simulink model "LugRStEnCtrl"  (R2018b)
settings: Solver=FixedStepDiscrete  StartTime=0.0  StopTime=10.0  FixedStep=0.01  RelTol=1e-3
undefined symbols (not defined in the file or in its folder): data, ThdRwRtStBkReclnEn_Clear, ThdRwRtStBkReclnEn_Set, ThdRwRtStCshnFldEn_Clear, ThdRwRtStCshnFldEn_Set, ThdRwRtStFwdBkwdEn_Clear, ThdRwRtStFwdBkwdEn_Set
libraries: simulink x1
settings Model: Creator=sn2xws  LastModifiedBy=sn2xws
settings DataIOCC: SaveFormat=StructureWithTime
settings OptimizationCC: DefaultParameterBehavior=Inlined  EnhancedBackFolding=on  PassReuseOutputArgsAs=Individual arguments  ZeroExternalMemoryAtStartup=off  ZeroInternalMemoryAtStartup=off  OptimizeBlockOrder=speed  DifferentSizesBufferReuse=on  OptimizationCustomize=off
settings DebuggingCC: ParameterTunabilityLossMsg=error
settings ModelReferenceCC: ModelReferenceNumInstancesAllowed=Single
settings SFSimCC: MATLABDynamicMemAlloc=off
settings RTWCC: SystemTargetFile=autosar.tlc  GenCodeOnly=on  TemplateMakefile=ert_default_tmf  Description=AUTOSAR  GenerateReport=on  IncludeHyperlinkInReport=on  LaunchReport=on  GenerateTraceInfo=on  GenerateTraceReport=on  GenerateTraceReportSl=on  GenerateTraceReportSf=on  GenerateTraceReportEml=on  GenerateCodeMetricsReport=on
settings CodeAppCC: ForceParamTrailComments=on  IgnoreCustomStorageClasses=off  OperatorAnnotations=on  SimulinkDataObjDesc=on  SFDataObjDesc=on  InsertBlockDesc=on
settings STFCustomTargetCC: TargetLangStandard=C99 (ISO)  MultiwordLength=256  ParMdlRefBuildCompliant=on  CompOptLevelCompliant=on  IncludeMdlTerminateFcn=off  CombineOutputUpdateFcns=on  SuppressErrorStatus=on  ERTCustomFileBanners=on  SupportNonFinite=off  SupportComplex=off  SupportContinuousTime=off  SupportNonInlinedSFcns=off  RemoveResetFunc=on  MATLABClassNameForMDSCustomization=Simulink.SoftwareTarget.ERTCustomization  AutosarCompliant=on  UseToolchainInfoCompliant=on  LookupTableObjectStructAxisOrder=2,1,3,4,...  LUTObjectStructOrderEvenSpacing=Size,Table,Breakpoints  SystemTargetFile=autosar.tlc
settings ERTTargetCC: TargetLangStandard=C99 (ISO)  ConcurrentExecutionCompliant=off  IncludeMdlTerminateFcn=off  SuppressErrorStatus=on  SupportNonFinite=off  SupportComplex=off  ModelStepFunctionPrototypeControlCompliant=off  CPPClassGenCompliant=off  AutosarCompliant=on  LookupTableObjectStructAxisOrder=2,1,3,4,...  LUTObjectStructOrderEvenSpacing=Size,Table,Breakpoints  InlinedParameterPlacement=NonHierarchical  ERTCustomFileTemplate=example_file_process.tlc  ERTFilePackagingFormat=Compact

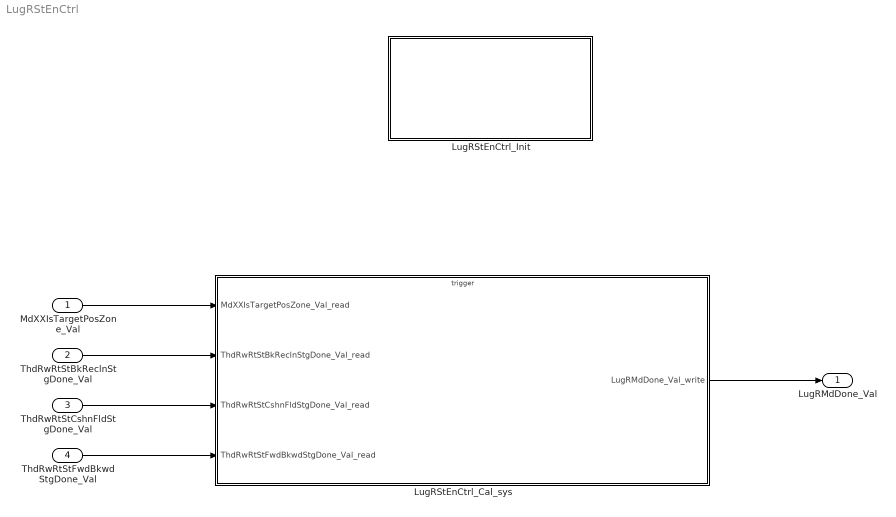
== system LugRStEnCtrl ==
  MdXXIsTargetPosZone_Val : Inport  OutDataTypeStr=uint32  PortDimensions=1
  ThdRwRtStBkReclnStgDone_Val : Inport  Port=2  OutDataTypeStr=boolean  PortDimensions=1
  ThdRwRtStCshnFldStgDone_Val : Inport  Port=3  OutDataTypeStr=boolean  PortDimensions=1
  ThdRwRtStFwdBkwdStgDone_Val : Inport  Port=4  OutDataTypeStr=boolean  PortDimensions=1
  LugRStEnCtrl_Cal_sys : Subsystem
  LugRStEnCtrl_Init : Subsystem
  LugRMdDone_Val : Outport  OutDataTypeStr=uint8  PortDimensions=1
  wires:
  MdXXIsTargetPosZone_Val/1 -> LugRStEnCtrl_Cal_sys/1(MdXXIsTargetPosZone_Val_read)
  ThdRwRtStBkReclnStgDone_Val/1 -> LugRStEnCtrl_Cal_sys/2(ThdRwRtStBkReclnStgDone_Val_read)
  ThdRwRtStCshnFldStgDone_Val/1 -> LugRStEnCtrl_Cal_sys/3(ThdRwRtStCshnFldStgDone_Val_read)
  ThdRwRtStFwdBkwdStgDone_Val/1 -> LugRStEnCtrl_Cal_sys/4(ThdRwRtStFwdBkwdStgDone_Val_read)
  LugRStEnCtrl_Cal_sys/1(LugRMdDone_Val_write) -> LugRMdDone_Val/1

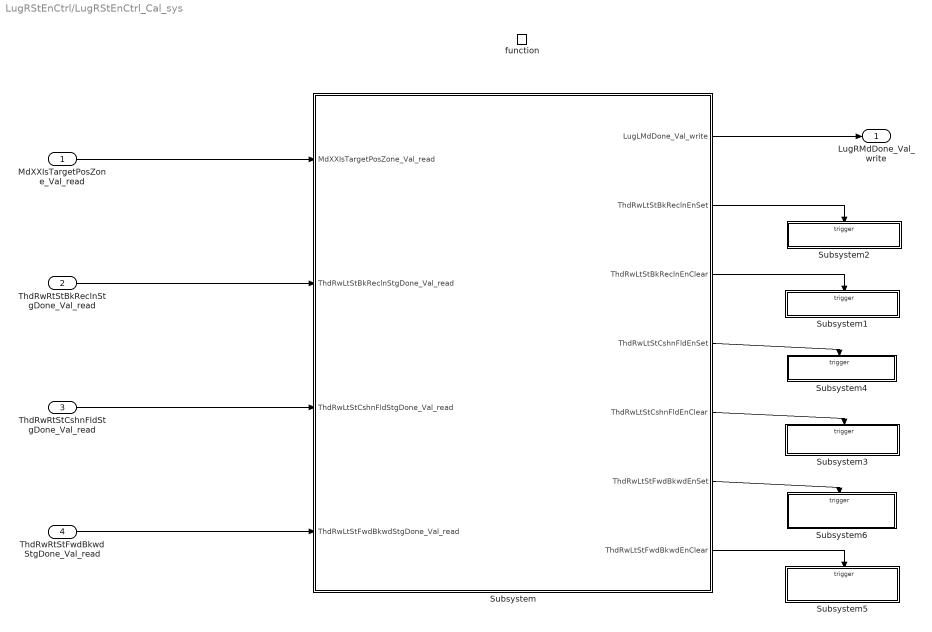
== system LugRStEnCtrl/LugRStEnCtrl_Cal_sys ==
  MdXXIsTargetPosZone_Val_read : Inport
  ThdRwRtStBkReclnStgDone_Val_read : Inport  Port=2
  ThdRwRtStCshnFldStgDone_Val_read : Inport  Port=3
  ThdRwRtStFwdBkwdStgDone_Val_read : Inport  Port=4
  function : TriggerPort  TriggerType=function-call  IsSimulinkFunction=on  FunctionName=LugRStEnCtrl_Cal  VariantControl=(inherit)
  Subsystem : Subsystem
  Subsystem1 : Subsystem
  Subsystem2 : Subsystem
  Subsystem3 : Subsystem
  Subsystem4 : Subsystem
  Subsystem5 : Subsystem
  Subsystem6 : Subsystem
  LugRMdDone_Val_write : Outport
      settings: EnsureOutportIsVirtual=on
  wires:
  Subsystem/7(ThdRwLtStFwdBkwdEnClear) -> Subsystem5/Trigger
  Subsystem/6(ThdRwLtStFwdBkwdEnSet) -> Subsystem6/Trigger
  Subsystem/4(ThdRwLtStCshnFldEnSet) -> Subsystem4/Trigger
  Subsystem/3(ThdRwLtStBkReclnEnClear) -> Subsystem1/Trigger
  Subsystem/2(ThdRwLtStBkReclnEnSet) -> Subsystem2/Trigger
  Subsystem/5(ThdRwLtStCshnFldEnClear) -> Subsystem3/Trigger
  Subsystem/1(LugLMdDone_Val_write) -> LugRMdDone_Val_write/1
  MdXXIsTargetPosZone_Val_read/1 -> Subsystem/1(MdXXIsTargetPosZone_Val_read)
  ThdRwRtStBkReclnStgDone_Val_read/1 -> Subsystem/2(ThdRwLtStBkReclnStgDone_Val_read)
  ThdRwRtStFwdBkwdStgDone_Val_read/1 -> Subsystem/4(ThdRwLtStFwdBkwdStgDone_Val_read)
  ThdRwRtStCshnFldStgDone_Val_read/1 -> Subsystem/3(ThdRwLtStCshnFldStgDone_Val_read)

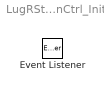
== system LugRStEnCtrl/LugRStEnCtrl_Init ==
  Event Listener : EventListener  EventName=reset

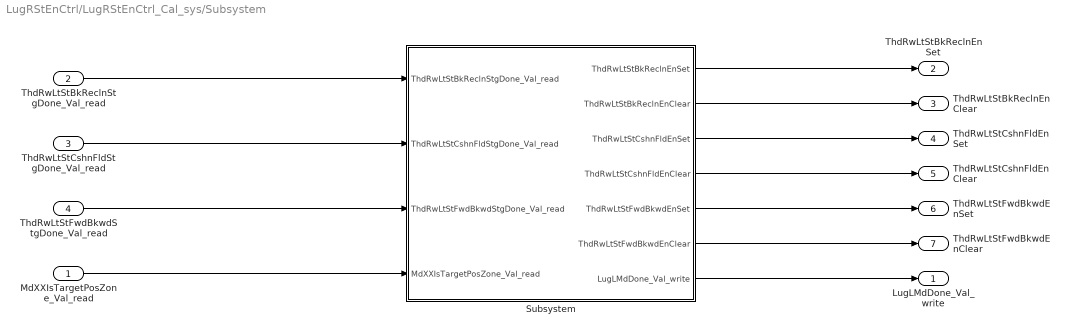
== system LugRStEnCtrl/LugRStEnCtrl_Cal_sys/Subsystem ==
  MdXXIsTargetPosZone_Val_read : Inport
  ThdRwLtStBkReclnStgDone_Val_read : Inport  Port=2
  ThdRwLtStCshnFldStgDone_Val_read : Inport  Port=3
  ThdRwLtStFwdBkwdStgDone_Val_read : Inport  Port=4
  Subsystem : Subsystem
  LugLMdDone_Val_write : Outport
      settings: EnsureOutportIsVirtual=on
  ThdRwLtStBkReclnEnSet : Outport  Port=2
  ThdRwLtStBkReclnEnClear : Outport  Port=3
  ThdRwLtStCshnFldEnSet : Outport  Port=4
  ThdRwLtStCshnFldEnClear : Outport  Port=5
  ThdRwLtStFwdBkwdEnSet : Outport  Port=6
  ThdRwLtStFwdBkwdEnClear : Outport  Port=7
  wires:
  Subsystem/7(LugLMdDone_Val_write) -> LugLMdDone_Val_write/1
  ThdRwLtStBkReclnStgDone_Val_read/1 -> Subsystem/1(ThdRwLtStBkReclnStgDone_Val_read)
  ThdRwLtStCshnFldStgDone_Val_read/1 -> Subsystem/2(ThdRwLtStCshnFldStgDone_Val_read)
  ThdRwLtStFwdBkwdStgDone_Val_read/1 -> Subsystem/3(ThdRwLtStFwdBkwdStgDone_Val_read)
  Subsystem/1(ThdRwLtStBkReclnEnSet) -> ThdRwLtStBkReclnEnSet/1
  Subsystem/2(ThdRwLtStBkReclnEnClear) -> ThdRwLtStBkReclnEnClear/1
  Subsystem/3(ThdRwLtStCshnFldEnSet) -> ThdRwLtStCshnFldEnSet/1
  Subsystem/4(ThdRwLtStCshnFldEnClear) -> ThdRwLtStCshnFldEnClear/1
  Subsystem/5(ThdRwLtStFwdBkwdEnSet) -> ThdRwLtStFwdBkwdEnSet/1
  Subsystem/6(ThdRwLtStFwdBkwdEnClear) -> ThdRwLtStFwdBkwdEnClear/1
  MdXXIsTargetPosZone_Val_read/1 -> Subsystem/4(MdXXIsTargetPosZone_Val_read)

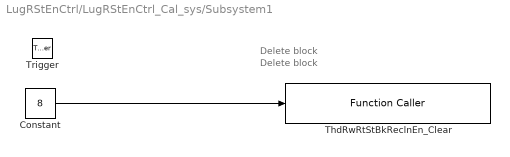
== system LugRStEnCtrl/LugRStEnCtrl_Cal_sys/Subsystem1 ==
  note: Delete block
  note: Delete block
  Trigger : TriggerPort  TriggerType=function-call  VariantControl=Variant  PortDimensions=1
  Constant : Constant  Value=8  OutDataTypeStr=uint8
  ThdRwRtStBkReclnEn_Clear : FunctionCaller  FunctionPrototype=ThdRwRtStBkReclnEn_Clear(data)  InputArgumentSpecifications=uint8(1)
  wires:
  Constant/1 -> ThdRwRtStBkReclnEn_Clear/1

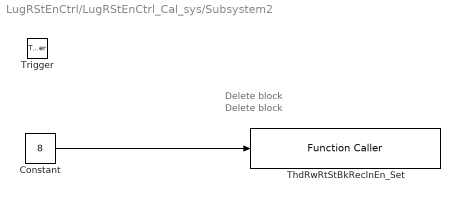
== system LugRStEnCtrl/LugRStEnCtrl_Cal_sys/Subsystem2 ==
  note: Delete block
  note: Delete block
  Trigger : TriggerPort  TriggerType=function-call  VariantControl=Variant  PortDimensions=1
  Constant : Constant  Value=8  OutDataTypeStr=uint8
  ThdRwRtStBkReclnEn_Set : FunctionCaller  FunctionPrototype=ThdRwRtStBkReclnEn_Set(data)  InputArgumentSpecifications=uint8(1)
  wires:
  Constant/1 -> ThdRwRtStBkReclnEn_Set/1

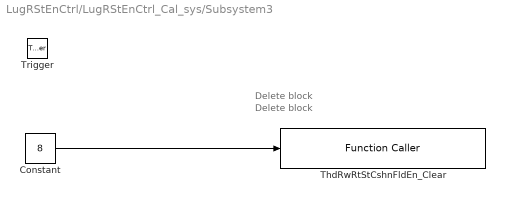
== system LugRStEnCtrl/LugRStEnCtrl_Cal_sys/Subsystem3 ==
  note: Delete block
  note: Delete block
  Trigger : TriggerPort  TriggerType=function-call  VariantControl=Variant  PortDimensions=1
  Constant : Constant  Value=8  OutDataTypeStr=uint8
  ThdRwRtStCshnFldEn_Clear : FunctionCaller  FunctionPrototype=ThdRwRtStCshnFldEn_Clear(data)  InputArgumentSpecifications=uint8(1)
  wires:
  Constant/1 -> ThdRwRtStCshnFldEn_Clear/1

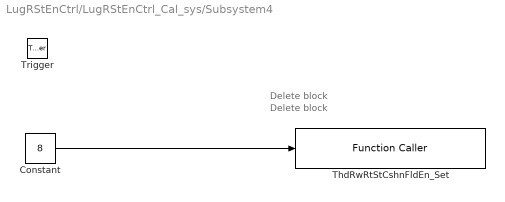
== system LugRStEnCtrl/LugRStEnCtrl_Cal_sys/Subsystem4 ==
  note: Delete block
  note: Delete block
  Trigger : TriggerPort  TriggerType=function-call  VariantControl=Variant  PortDimensions=1
  Constant : Constant  Value=8  OutDataTypeStr=uint8
  ThdRwRtStCshnFldEn_Set : FunctionCaller  FunctionPrototype=ThdRwRtStCshnFldEn_Set(data)  InputArgumentSpecifications=uint8(1)
  wires:
  Constant/1 -> ThdRwRtStCshnFldEn_Set/1

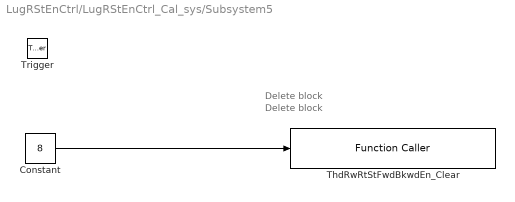
== system LugRStEnCtrl/LugRStEnCtrl_Cal_sys/Subsystem5 ==
  note: Delete block
  note: Delete block
  Trigger : TriggerPort  TriggerType=function-call  VariantControl=Variant  PortDimensions=1
  Constant : Constant  Value=8  OutDataTypeStr=uint8
  ThdRwRtStFwdBkwdEn_Clear : FunctionCaller  FunctionPrototype=ThdRwRtStFwdBkwdEn_Clear(data)  InputArgumentSpecifications=uint8(1)
  wires:
  Constant/1 -> ThdRwRtStFwdBkwdEn_Clear/1

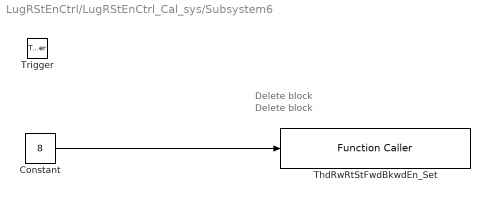
== system LugRStEnCtrl/LugRStEnCtrl_Cal_sys/Subsystem6 ==
  note: Delete block
  note: Delete block
  Trigger : TriggerPort  TriggerType=function-call  VariantControl=Variant  PortDimensions=1
  Constant : Constant  Value=8  OutDataTypeStr=uint8
  ThdRwRtStFwdBkwdEn_Set : FunctionCaller  FunctionPrototype=ThdRwRtStFwdBkwdEn_Set(data)  InputArgumentSpecifications=uint8(1)
  wires:
  Constant/1 -> ThdRwRtStFwdBkwdEn_Set/1

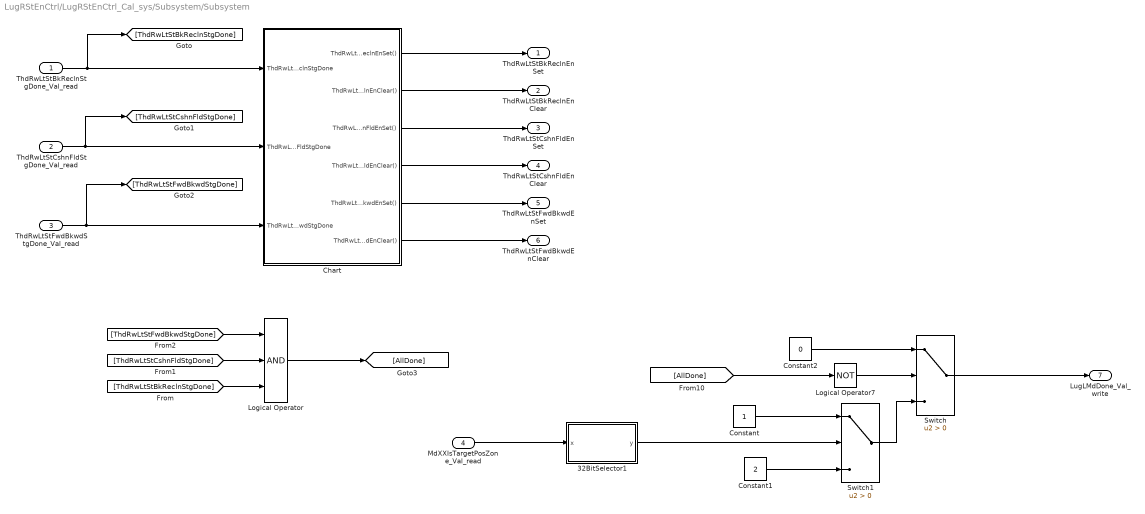
== system LugRStEnCtrl/LugRStEnCtrl_Cal_sys/Subsystem/Subsystem ==
  ThdRwLtStBkReclnStgDone_Val_read : Inport
  ThdRwLtStCshnFldStgDone_Val_read : Inport  Port=2
  ThdRwLtStFwdBkwdStgDone_Val_read : Inport  Port=3
  MdXXIsTargetPosZone_Val_read : Inport  Port=4
  32BitSelector1 : Subsystem  mask(32 Bit Selector){BitNum=8}
      mask prompts: BitNum "Select Bit Number"
      mask help: Allows selection of a particular bit (0-31) out of a packed word up to 32 bits long. Output will be true if the bit number selected via the mask parameter is equal to one.
      mask TypeOptions BitNum: 0 | 1 | 2 | 3 | 4 | 5 | 6 | 7 | 8 | 9 | 10 | 11 | 12 | 13 | 14 | 15 | 16 | 17 | 18 | 19 | 20 | 21 | 22 | 23 | 24 | 25 | 26 | 27 | 28 | 29 | 30 | 31
      mask Display:
      | text(0.5, 0.8,'BIT','horizontalAlignment','center')
      | text(0.5, 0.5,'SELECTOR','horizontalAlignment','center')
      | text(0.5, 0.2,['-- Bit ',char(get_param(gcb,'BitNum')),' --'],'horizontalAlignment','center')
  Chart : Stateflow chart  TreatAsAtomicUnit=on
  Constant : Constant  OutDataTypeStr=uint8
  Constant1 : Constant  Value=2  OutDataTypeStr=uint8
  Constant2 : Constant  Value=0  OutDataTypeStr=uint8
  Logical Operator : Logic  Inputs=3  AllPortsSameDT=off  OutDataTypeStr=boolean
  Logical Operator7 : Logic  Operator=NOT  AllPortsSameDT=off  OutDataTypeStr=boolean
  Switch : Switch  Criteria=u2 > Threshold
  Switch1 : Switch  Criteria=u2 > Threshold
  ThdRwLtStBkReclnEnSet : Outport
  ThdRwLtStBkReclnEnClear : Outport  Port=2
  ThdRwLtStCshnFldEnSet : Outport  Port=3
  ThdRwLtStCshnFldEnClear : Outport  Port=4
  ThdRwLtStFwdBkwdEnSet : Outport  Port=5
  ThdRwLtStFwdBkwdEnClear : Outport  Port=6
  LugLMdDone_Val_write : Outport  Port=7
      settings: EnsureOutportIsVirtual=on
  wires:
  Chart/1(ThdRwLtStBkReclnEnSet()) -> ThdRwLtStBkReclnEnSet/1
  Chart/2(ThdRwLtStBkReclnEnClear()) -> ThdRwLtStBkReclnEnClear/1
  Chart/3(ThdRwLtStCshnFldEnSet()) -> ThdRwLtStCshnFldEnSet/1
  Chart/4(ThdRwLtStCshnFldEnClear()) -> ThdRwLtStCshnFldEnClear/1
  Chart/5(ThdRwLtStFwdBkwdEnSet()) -> ThdRwLtStFwdBkwdEnSet/1
  Chart/6(ThdRwLtStFwdBkwdEnClear()) -> ThdRwLtStFwdBkwdEnClear/1
  MdXXIsTargetPosZone_Val_read/1 -> 32BitSelector1/1(x)
  [ThdRwLtStBkReclnStgDone] -> Logical Operator/3
  [ThdRwLtStFwdBkwdStgDone] -> Logical Operator/1
  [ThdRwLtStCshnFldStgDone] -> Logical Operator/2
  Logical Operator/1 -> [AllDone]
  Switch1/1 -> Switch/3
  Switch/1 -> LugLMdDone_Val_write/1
  ThdRwLtStBkReclnStgDone_Val_read/1 -> [ThdRwLtStBkReclnStgDone], Chart/1(ThdRwLtStBkReclnStgDone)
  ThdRwLtStCshnFldStgDone_Val_read/1 -> [ThdRwLtStCshnFldStgDone], Chart/2(ThdRwLtStCshnFldStgDone)
  ThdRwLtStFwdBkwdStgDone_Val_read/1 -> [ThdRwLtStFwdBkwdStgDone], Chart/3(ThdRwLtStFwdBkwdStgDone)
  Constant2/1 -> Switch/1
  Constant1/1 -> Switch1/3
  Constant/1 -> Switch1/1
  [AllDone] -> Logical Operator7/1
  Logical Operator7/1 -> Switch/2
  32BitSelector1/1(y) -> Switch1/2

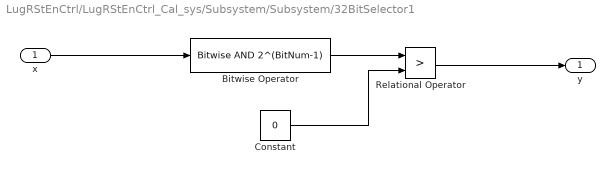
== system LugRStEnCtrl/LugRStEnCtrl_Cal_sys/Subsystem/Subsystem/32BitSelector1 ==
  x : Inport
  Bitwise Operator : simulink/Logic and Bit Operations/Bitwise Operator  logicop=AND  UseBitMask=on  BitMask=2^(BitNum-1)  BitMaskRealWorld=Stored Integer
  Constant : Constant  Value=0  OutDataTypeStr=uint32
  Relational Operator : RelationalOperator  Operator=>  OutDataTypeStr=boolean  RndMeth=Simplest
  y : Outport
  wires:
  Relational Operator/1 -> y/1
  Constant/1 -> Relational Operator/2
  x/1 -> Bitwise Operator/1
  Bitwise Operator/1 -> Relational Operator/1

== stateflow chart LugRStEnCtrl/LugRStEnCtrl_Cal_sys/Subsystem/Subsystem/Chart ==
  (default) -> (junction 9)
  (junction 9) -> (junction 49) [order 1] : [ThdRwLtStBkReclnStgDone]
  (junction 9) -> (junction 53) [order 2] : {
      | ThdRwLtStBkReclnEnSet;
      | }
  (junction 49) -> (junction 51) : {
      | ThdRwLtStBkReclnEnClear;
      | }
  (junction 51) -> (junction 53)
  (junction 53) -> (junction 121)
  (junction 121) -> (junction 122) [order 1] : [ThdRwLtStCshnFldStgDone]
  (junction 121) -> (junction 126) [order 2] : {
      | ThdRwLtStCshnFldEnSet;
      | }
  (junction 122) -> (junction 124) : {
      | ThdRwLtStCshnFldEnClear;
      | }
  (junction 124) -> (junction 126)
  (junction 126) -> (junction 58)
  (junction 58) -> (junction 60) [order 1] : [(ThdRwLtStBkReclnStgDone&&ThdRwLtStCshnFldStgDone)]
  (junction 60) -> (junction 62) [order 1] : [ThdRwLtStFwdBkwdStgDone]
  (junction 58) -> (junction 7) [order 2] : {
      | ThdRwLtStFwdBkwdEnClear;
      | }
  (junction 60) -> (junction 66) [order 2] : {
      | ThdRwLtStFwdBkwdEnSet;
      | }
  (junction 62) -> (junction 64) : {
      | ThdRwLtStFwdBkwdEnClear;
      | }
  (junction 66) -> (junction 7)
  (junction 64) -> (junction 66)
  data: ThdRwLtStBkReclnStgDone input boolean; ThdRwLtStCshnFldStgDone input boolean; ThdRwLtStFwdBkwdStgDone input boolean
  events: ThdRwLtStBkReclnEnSet output FUNCTION_CALL_EVENT; ThdRwLtStBkReclnEnClear output FUNCTION_CALL_EVENT; ThdRwLtStCshnFldEnSet output FUNCTION_CALL_EVENT; ThdRwLtStCshnFldEnClear output FUNCTION_CALL_EVENT; ThdRwLtStFwdBkwdEnSet output FUNCTION_CALL_EVENT; ThdRwLtStFwdBkwdEnClear output FUNCTION_CALL_EVENT
